simulink model "model_buck_boost"  (R2022b)
settings: Solver=ode45  StartTime=0.0  StopTime=0.1  RelTol=1e-3  EnableMultiTasking=on
values from neighbouring files (symbols this model uses):
  C = 22e-6    (= 2.2e-05)    [loop_buck_boost.m]    (also in loop_cuk.m; var_buck_boost.m; var_cuk.m)
  closedLoop = 0    [loop_buck_boost.m]    (also in var_buck_boost.m = 1)
  dD_delta = 0.1    [loop_buck_boost.m]    (also in var_buck_boost.m)
  dD_med = 0.6    [loop_buck_boost.m]    (also in var_buck_boost.m; var_cuk.m = 0.5)
  kd = 0    [loop_buck_boost.m]    (also in var_buck_boost.m = 0.4)
  ki = 0    [loop_buck_boost.m]    (also in var_buck_boost.m = 8)
  kp = 10    [loop_buck_boost.m]    (also in var_buck_boost.m)
  L = 1e-3    (= 0.001)    [loop_buck_boost.m]    (also in loop_cuk.m = 4.7e-05; var_buck_boost.m; var_cuk.m = 4.7e-05)
  LL = 5e-3    (= 0.005)    [loop_buck_boost.m]    (also in loop_cuk.m = 0.001; sim_buck_boost.m = LLs(i); sim_cuk.m = LLs(i); var_buck_boost.m)
  omega = 100    [loop_buck_boost.m]    (also in var_buck_boost.m)
  omega_chav = 100    [var_buck_boost.m]
  r_delta = 10    [loop_buck_boost.m]    (also in var_buck_boost.m)
  r_med = 30    [loop_buck_boost.m]    (also in var_buck_boost.m)
  rc = 150e-3    (= 0.15)    [loop_buck_boost.m]    (also in var_buck_boost.m)
  rL = 20e-3    (= 0.02)    [loop_buck_boost.m]    (also in loop_cuk.m = 0.03; var_buck_boost.m; var_cuk.m = 0.03)
  RL = 5    [loop_buck_boost.m]    (also in sim_buck_boost.m = RLs(i); sim_cuk.m = RLs(i); var_buck_boost.m)
  rs = 25e-3    (= 0.025)    [loop_buck_boost.m]    (also in loop_cuk.m = 0.03; var_buck_boost.m; var_cuk.m = 0.03)
libraries: slpidlib x1
settings Model: Creator=11802972  LastModifiedBy=andre
settings SolverCC: AlgebraicLoopSolver=TrustRegion
settings DataIOCC: LimitDataPoints=on  SaveFormat=Array  ReturnWorkspaceOutputs=off
settings OptimizationCC: LifeSpan=inf
settings DebuggingCC: UnconnectedInputMsg=warning  UnconnectedOutputMsg=warning  UnconnectedLineMsg=warning  SFUnexpectedBacktrackingDiag=warning  SFNoUnconditionalDefaultTransitionDiag=warning  SFExecutionAtInitializationDiag=none  SFMachineParentedDataDiag=warning  ArithmeticOperatorsInVariantConditions=warning
settings HardwareCC: ProdBitPerPointer=32  ProdBitPerSizeT=32  ProdBitPerPtrDiffT=32  ProdLargestAtomicFloat=None  ProdIntDivRoundTo=Undefined  ProdEndianess=Unspecified  ProdWordSize=32  ProdHWDeviceType=32-bit Generic
settings ModelReferenceCC: PropagateSignalLabelsOutOfModel=off
settings SFSimCC: SimUseLocalCustomCode=off  CustomCodeUndefinedFunction=UseInterfaceOnly
settings RTWCC: RTWUseLocalCustomCode=off
settings CodeAppCC: StateflowObjectComments=on
settings GRTTargetCC: TargetLangStandard=C89/C90 (ANSI)
settings ConfigComp: CovMetricSettings=dw  CovSaveCumulativeToWorkspaceVar=on  CovSaveSingleToWorkspaceVar=on  CovExternalEMLEnable=off

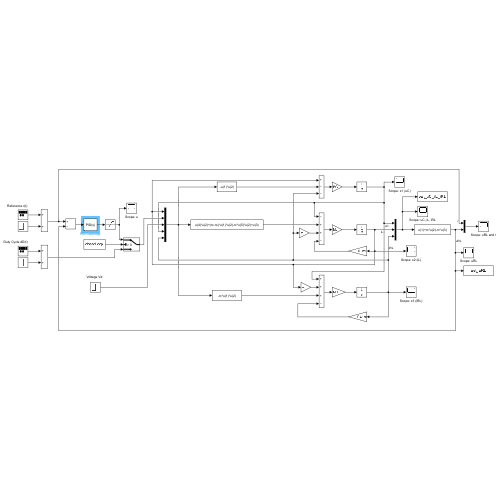
[thumbnail: Simulink's stored preview of the top-level diagram]
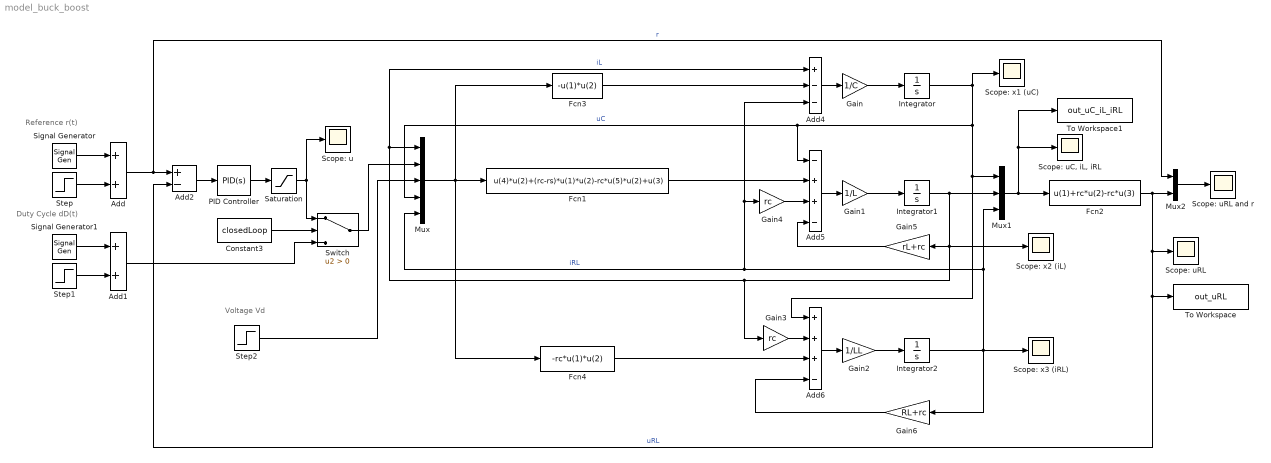
== system model_buck_boost ==
  note: Voltage Vd
  note: Duty Cycle dD(t)
  note: Reference r(t)
  Add : Sum
  Add1 : Sum
  Add2 : Sum  Inputs=+-
  Add4 : Sum  Inputs=+--
  Add5 : Sum  Inputs=-++-
  Add6 : Sum  Inputs=+++-
  Constant3 : Constant  Value=closedLoop
  Fcn1 : Fcn  Expr=u(4)*u(2)+(rc-rs)*u(1)*u(2)-rc*u(5)*u(2)+u(3)
  Fcn2 : Fcn  Expr=u(1)+rc*u(2)-rc*u(3)
  Fcn3 : Fcn  Expr=-u(1)*u(2)
  Fcn4 : Fcn  Expr=-rc*u(1)*u(2)
  Gain : Gain  Gain=1/C
  Gain1 : Gain  Gain=1/L
  Gain2 : Gain  Gain=1/LL
  Gain3 : Gain  Gain=rc
  Gain4 : Gain  Gain=rc
  Gain5 : Gain  Gain=rL+rc
  Gain6 : Gain  Gain=RL+rc
  Integrator : Integrator
  Integrator1 : Integrator
  Integrator2 : Integrator
  Mux : Mux  Inputs=5
  Mux1 : Mux  Inputs=3
  Mux2 : Mux  Inputs=2
  PID Controller : slpidlib/PID Controller  Controller=PID  Form=Parallel  TimeDomain=Continuous-time  UseExternalTs=off  SampleTime=-1  IntegratorMethod=Forward Euler  FilterMethod=Forward Euler  ControllerParametersSource=internal  P=kp  I=ki  UseKiTs=off  D=kd  N=100  UseFilter=on  TunerSelectOption=Transfer Function Based (PID Tuner App)  InitialConditionSource=internal  InitialConditionForIntegrator=0  InitialConditionForFilter=0  DifferentiatorICPrevScaledInput=0  ExternalReset=none  TrackingMode=off  Kt=1  LimitOutput=off  SatLimitsSource=internal  UpperSaturationLimit=inf  LowerSaturationLimit=-inf  LinearizeAsGain=on  AntiWindupMode=none  Kb=1  LimitIntegrator=off  UpperIntegratorSaturationLimit=inf  LowerIntegratorSaturationLimit=-inf  POutMin=[]  POutMax=[]  IOutMin=[]  IOutMax=[]  DOutMin=[]  DOutMax=[]  NOutMin=[]  NOutMax=[]  SumOutMin=[]  SumOutMax=[]  SaturationOutMin=[]  SaturationOutMax=[]  PParamMin=[]  PParamMax=[]  IParamMin=[]  IParamMax=[]  DParamMin=[]  DParamMax=[]  NParamMin=[]  NParamMax=[]  KbParamMin=[]  KbParamMax=[]  KtParamMin=[]  KtParamMax=[]  KbOutMin=[]  KbOutMax=[]  KtOutMin=[]  KtOutMax=[]  IntegratorOutMin=[]  IntegratorOutMax=[]  FilterOutMin=[]  FilterOutMax=[]  SumI1OutMin=[]  SumI1OutMax=[]  SumI2OutMin=[]  SumI2OutMax=[]  SumI3OutMin=[]  SumI3OutMax=[]  SumI4OutMin=[]  SumI4OutMax=[]  SumDOutMin=[]  SumDOutMax=[]  DifferentiatorOutMin=[]  DifferentiatorOutMax=[]  FilterDiffOutCoefMin=[]  FilterDiffOutCoefMax=[]  ReciprocalOutMin=[]  ReciprocalOutMax=[]  SumDenOutMin=[]  SumDenOutMax=[]  SumNumOutMin=[]  SumNumOutMax=[]  DivideOutMin=[]  DivideOutMax=[]  UdiffTsProdOutMin=[]  UdiffTsProdOutMax=[]  NTsProdOutMin=[]  NTsProdOutMax=[]  UintegralTsProdOutMin=[]  UintegralTsProdOutMax=[]  UngainTsProdOutMin=[]  UngainTsProdOutMax=[]  ClampingZeroOutDataTypeStr=Inherit: Inherit via back propagation  ClampingZeroOutMin=[]  ClampingZeroOutMax=[]  FilterDenConstantOutDataTypeStr=Inherit: Inherit via back propagation  FilterDenConstantOutMin=[]  FilterDenConstantOutMax=[]  PCopyOutDataTypeStr=Inherit: Inherit via back propagation  PCopyOutMin=[]  PCopyOutMax=[]  NCopyOutDataTypeStr=Inherit: Inherit via back propagation  NCopyOutMin=[]  NCopyOutMax=[]  IntegratorContinuousStateAttributes=''  IntegratorStateMustResolveToSignalObject=off  IntegratorRTWStateStorageClass=Auto  FilterContinuousStateAttributes=''  FilterStateMustResolveToSignalObject=off  FilterRTWStateStorageClass=Auto  ParallelPVariant=InternalParameters  IdealPVariant=Disabled  IVariant=InternalParameters  DVariant=InternalParameters  IntegratorVariant=Continuous  SatVariant=Disabled  AWVariant=Passthrough  PCopyVariant=Disabled  TRVariant=Disabled  FdbkBlocksVariant=Forward  IdealPFdbkVariant=Disabled  SatFdbkVariant=Disabled  DerivativeFilterVariant=ContFilter  NVariant=InternalParameters  NCopyVariant=Disabled  FilterICVariant=InternalICsFilter  IntegratorICVariant=InternalICs  ExternalResetVariant=Disabled  TRSumVariant=Passthrough  SumFdbkVariant=Disabled  SumVariant=Sum_PID  TsampFilterVariant=InternalTs  TsampNgainVariant=Passthrough  TsampIntegralVariant=Passthrough  ExternalSaturationOutDataTypeStr=Inherit: Same as second input
  Saturation : Saturate  UpperLimit=1  LowerLimit=0
  Scope: u : Scope
  "Scope: uC, iL, iRL" : Scope
  Scope: uRL : Scope
  Scope: uRL and r : Scope
  Scope: x1 (uC) : Scope
  Scope: x2 (iL) : Scope
  Scope: x3 (iRL) : Scope
  Signal Generator : SignalGenerator  WaveForm=square  Amplitude=-r_delta  Frequency=omega  Units=rad/sec
  Signal Generator1 : SignalGenerator  WaveForm=square  Amplitude=-dD_delta  Frequency=omega_chav  Units=rad/sec
  Step : Step  Time=0  After=r_med  SampleTime=0
  Step1 : Step  Time=0  After=dD_med  SampleTime=0
  Step2 : Step  Time=0  After=10  SampleTime=0
  Switch : Switch  Criteria=u2 > Threshold  SaturateOnIntegerOverflow=off  InputSameDT=off
  To Workspace : ToWorkspace  VariableName=out_uRL  SaveFormat=Timeseries  SampleTime=-1
  To Workspace1 : ToWorkspace  VariableName=out_uC_iL_iRL  SaveFormat=Timeseries  SampleTime=-1
  wires:
  Signal Generator/1 -> Add/1
  Signal Generator1/1 -> Add1/1
  Add/1 -> Mux2/1, Add2/1  "r"
  Add2/1 -> PID Controller/1
  PID Controller/1 -> Saturation/1
  Step2/1 -> Mux/3
  Mux/1 -> Fcn4/1, Fcn3/1, Fcn1/1
  Fcn3/1 -> Add4/2
  Fcn1/1 -> Add5/2
  Add4/1 -> Gain/1
  Add5/1 -> Gain1/1
  Fcn4/1 -> Add6/3
  Add6/1 -> Gain2/1
  Gain3/1 -> Add6/2
  Gain4/1 -> Add5/3
  Gain/1 -> Integrator/1
  Gain1/1 -> Integrator1/1
  Gain2/1 -> Integrator2/1
  Integrator/1 -> Mux1/1, Add6/1, Add5/1, Mux/4, Scope: x1 (uC)/1  "uC"
  Integrator1/1 -> Scope: x2 (iL)/1, Gain3/1, Add4/1, Mux/1, Gain5/1, Mux1/2  "iL"
  Mux1/1 -> To Workspace1/1, "Scope: uC, iL, iRL"/1, Fcn2/1
  Fcn2/1 -> Mux2/2, Scope: uRL/1, Add2/2, To Workspace/1  "uRL"
  Mux2/1 -> Scope: uRL and r/1
  Gain5/1 -> Add5/4
  Gain6/1 -> Add6/4
  Integrator2/1 -> Mux1/3, Add4/3, Gain4/1, Mux/5, Scope: x3 (iRL)/1, Gain6/1  "iRL"
  Step/1 -> Add/2
  Step1/1 -> Add1/2
  Add1/1 -> Switch/3
  Constant3/1 -> Switch/2
  Saturation/1 -> Switch/1, Scope: u/1
  Switch/1 -> Mux/2
